simulink subsystem "Robot_SubSystem"  (R2020b)
settings: Solver=VariableStepAuto  StartTime=0.0  StopTime=10.0  RelTol=1e-3
settings Model: Creator=umberto  LastModifiedBy=umberto

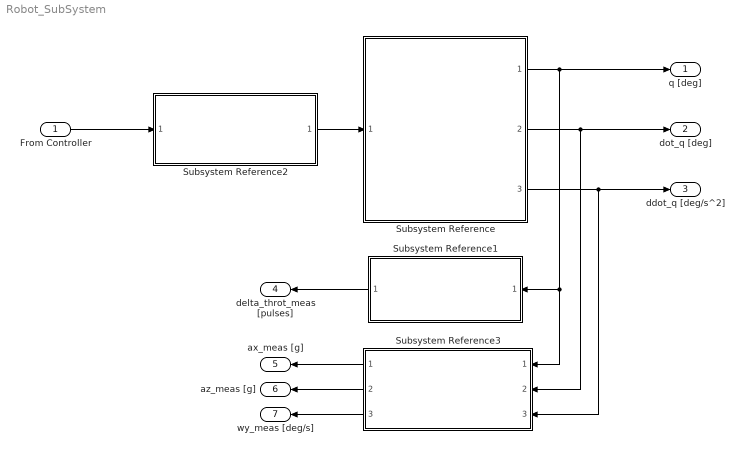
== system Robot_SubSystem ==
  From Controller : Inport
  Subsystem Reference : Subsystem  ReferencedSubsystem=Electromechanical_SubSystem
  Subsystem Reference1 : Subsystem  ReferencedSubsystem=Encoder_SubSystem
  Subsystem Reference2 : Subsystem  ReferencedSubsystem=VoltageDriver_SubSystem
  Subsystem Reference3 : Subsystem  ReferencedSubsystem=MPU_SubSystem
  q [deg] : Outport
  dot_q [deg] : Outport  Port=2
  ddot_q [deg/s^2] : Outport  Port=3
  delta_throt_meas [pulses] : Outport  Port=4
  ax_meas [g] : Outport  Port=5
  az_meas [g] : Outport  Port=6
  wy_meas [deg/s] : Outport  Port=7
  wires:
  Subsystem Reference2/1 -> Subsystem Reference/1
  Subsystem Reference/2 -> dot_q [deg]/1, Subsystem Reference3/2
  Subsystem Reference/3 -> ddot_q [deg/s^2]/1, Subsystem Reference3/3
  Subsystem Reference/1 -> q [deg]/1, Subsystem Reference3/1, Subsystem Reference1/1
  Subsystem Reference3/1 -> ax_meas [g]/1
  Subsystem Reference3/2 -> az_meas [g]/1
  Subsystem Reference3/3 -> wy_meas [deg/s]/1
  Subsystem Reference1/1 -> delta_throt_meas [pulses]/1
  From Controller/1 -> Subsystem Reference2/1
